simulink model "RRT_timer"  (Simulink 7.6)
settings: Solver=ode3  StartTime=0.0  StopTime=10.0  FixedStep=0.05  RelTol=1e-3
settings Model: Creator=Nikola  LastModifiedBy=Nikola
settings SimEventsCC: propDiagAttribOutput=1  propDiagFcnCallOutput=1  propDiagStatOutput=0

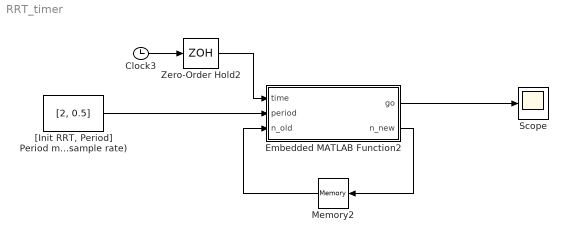
== system RRT_timer ==
  Clock3 : Clock
      settings: Decimation=10
  Embedded MATLAB Function2 : Stateflow chart  TreatAsAtomicUnit=on
  Memory2 : Memory  X0=1
  Scope : Scope
  Zero-Order Hold2 : ZeroOrderHold  SampleTime=0.05
  "[Init RRT, Period] Period must be multiple of 0.05 sec (global sample rate)" : Constant  Value=[2, 0.5]
  wires:
  Embedded MATLAB Function2/1(go) -> Scope/1
  Embedded MATLAB Function2/2(n_new) -> Memory2/1
  Memory2/1 -> Embedded MATLAB Function2/3(n_old)
  "[Init RRT, Period] Period must be multiple of 0.05 sec (global sample rate)"/1 -> Embedded MATLAB Function2/2(period)
  Clock3/1 -> Zero-Order Hold2/1
  Zero-Order Hold2/1 -> Embedded MATLAB Function2/1(time)

== matlab function Embedded MATLAB Function2 ==
  data: time input double; period input double; go output double; n_old input double; n_new output double
function [go,n_new] = tick_tock(time,period,n_old)
%#eml
t = time;
init_time = period(1);
T = period(2);

if t == T*n_old
    n_new = n_old + 1;
    if t >= init_time
        go = 1;
    else
        go = 0;
    end
else
    go = 0;
    n_new = n_old;
end
